simulink model "LUGOT"  (R2021a)
settings: Solver=FixedStepDiscrete  StartTime=0.0  StopTime=length(time_uwb)-1  FixedStep=Ts  MaxStep=Ts  RelTol=1e-3
values from neighbouring files (symbols this model uses):
  a = (vx .* ax + vy .* ay) ./ v    [relative_spd_vs_residual.m]    (also in smoothing_spline_fit.m)
  num_init_steps = uint8(3)    [main.m]
  outlier_threshold = standerd_deviation * 3.75 * 2 + 0.0    [main.m]
  Ts = 1.    (= 1)    [main.m]    (also in stateTransitionFcn_PF.m = 0.01)
undefined symbols (not defined in the file or in its folder): delta_h, Discrete, Time
libraries: sharedTrackingLibrary x9, simulink x6, dspstat3 x4, ctrlSharedLib x1
(part 1 of 2)
settings Model: Creator=bit202  LastModifiedBy=bit202
settings SolverCC: PositivePriorityOrder=on  AutoInsertRateTranBlk=on
settings DataIOCC: ReturnWorkspaceOutputs=off

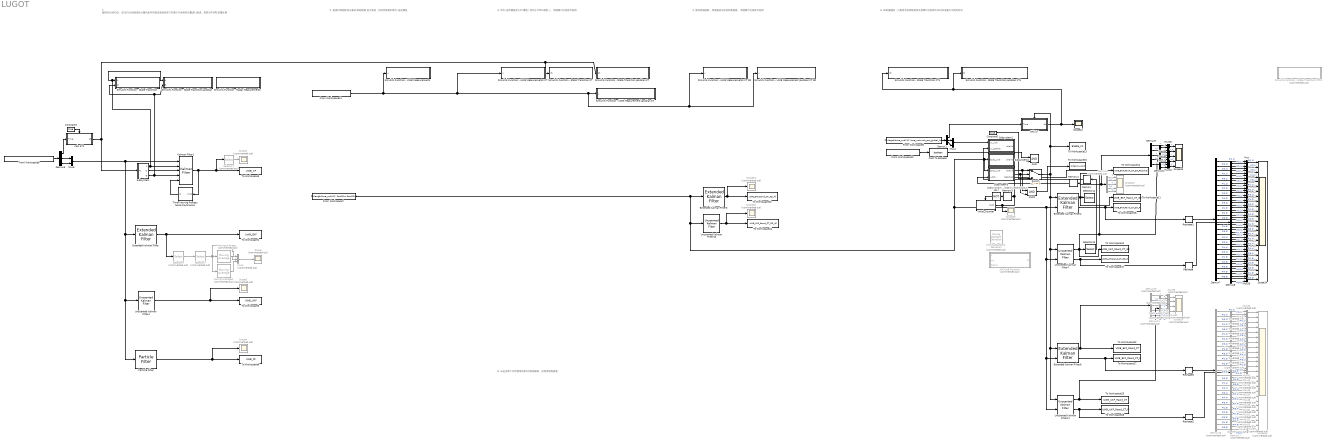
== system LUGOT ==
  note: 随着ΔT的变大，阈值可以考虑适当变大
  note: 1. 直接对分别对d1、d2进行分别滤波后计算的后车初始位姿坐标系下的笛卡尔坐标系位置进行滤波，把其当作GPS位置处理
  note: 2. 直接对观测标签与基站 原始距离 进行滤波，但仍然使用的是CV运动模型
  note: 3. 将CV运动模型改为CT模型（相当于CTRV模型）。
      | 观测雅可比矩阵不能用
  note: 4. 修改观测函数，考虑基站与标签的高度差。
      | 观测雅可比矩阵不能用
  note: 5. 异常值剔除，只是将状态转移矩阵及其雅可比矩阵的dt时间设置为不同的时间
  note: 6. 右边这两个仍然使用的是3的观测函数，没有考虑高度差
  AND : Logic  IconShape=distinctive  AllPortsSameDT=off  OutDataTypeStr=boolean
  AND1 : Logic  IconShape=distinctive  AllPortsSameDT=off  OutDataTypeStr=boolean
  Cast To Boolean : DataTypeConversion  OutDataTypeStr=boolean
  Constant1 : Constant  Value=true
  Constant3 : Constant  Value=true
  Demux1 : Demux  Outputs=3
  Demux10 : Demux  Outputs=5
  Demux11 : Demux  Commented=on  Outputs=5
  Demux16 : Demux  Commented=on  Outputs=25
  Demux17 : Demux  Commented=on  Outputs=25
  Demux18 : Demux  Commented=on  Outputs=5
  Demux3 : Demux  Outputs=3
  Demux4 : Demux  Commented=on  Outputs=5
  Demux7 : Demux  Outputs=25
  Demux8 : Demux  Outputs=25
  Demux9 : Demux  Outputs=5
  Extended Kalman Filter : sharedTrackingLibrary/Extended Kalman Filter  StateTransitionFcn=stateTransitionFcn  HasStateTransitionJacobianFcn=on  StateTransitionJacobianFcn=stateTransitionJacobianFcn  HasAdditiveProcessNoise=Nonadditive  ProcessNoise=[0.2 0; 0 0.2]  HasTimeVaryingProcessNoise=off  HasStateTransitionFcnExtraArgument=0  InitialState=[28; 0.001; 0.001; 0.001]  InitialStateCovariance=1  MeasurementFcn1=gpsMeasurementFcn  HasMeasurementJacobianFcn1=off  HasMeasurementEnablePort1=off  HasAdditiveMeasurementNoise1=Additive  MeasurementNoise1=[100 0; 0 100]  HasTimeVaryingMeasurementNoise1=off  HasMeasurementFcnExtraArgument1=0  MeasurementFcn2=myMeasurementFcn  HasMeasurementJacobianFcn2=off  HasMeasurementEnablePort2=off  HasAdditiveMeasurementNoise2=Additive  MeasurementNoise2=[0.0025 0; 0 0.0025]  HasTimeVaryingMeasurementNoise2=off  HasMeasurementFcnExtraArgument2=0  MeasurementFcn3=myMeasurementFcn  HasMeasurementJacobianFcn3=off  HasMeasurementEnablePort3=off  HasAdditiveMeasurementNoise3=Additive  MeasurementNoise3=1  HasTimeVaryingMeasurementNoise3=off  HasMeasurementFcnExtraArgument3=0  MeasurementFcn4=myMeasurementFcn  HasMeasurementJacobianFcn4=off  HasMeasurementEnablePort4=off  HasAdditiveMeasurementNoise4=Additive  MeasurementNoise4=1  HasTimeVaryingMeasurementNoise4=off  HasMeasurementFcnExtraArgument4=0  MeasurementFcn5=myMeasurementFcn  HasMeasurementJacobianFcn5=off  HasMeasurementEnablePort5=off  HasAdditiveMeasurementNoise5=Additive  MeasurementNoise5=1  HasTimeVaryingMeasurementNoise5=off  HasMeasurementFcnExtraArgument5=0  EnableMultirate=on  StateTransitionFcnSampleTime=Ts  MeasurementFcn1SampleTime=Ts  MeasurementFcn2SampleTime=1  MeasurementFcn3SampleTime=1  MeasurementFcn4SampleTime=1  MeasurementFcn5SampleTime=1  UseCurrentEstimator=on  OutputStateCovariance=off  DataType=double  SampleTime=0.01  NumberOfMeasurements=1
      settings: SourceProductBaseCode=CT,DR,TF,ID,LP,NV,AR,RO,RR,UV,VE
  Extended Kalman Filter2 : sharedTrackingLibrary/Extended Kalman Filter  StateTransitionFcn=stateTransitionCTEliminateFcn  HasStateTransitionJacobianFcn=on  StateTransitionJacobianFcn=stateTransitionJacobianCTFcn  HasAdditiveProcessNoise=Nonadditive  ProcessNoise=cov_process_noise  HasTimeVaryingProcessNoise=off  HasStateTransitionFcnExtraArgument=0  InitialState=init_state  InitialStateCovariance=0.5  MeasurementFcn1=uwbMeasurementCT3DFcn  HasMeasurementJacobianFcn1=off  MeasurementJacobianFcn1=uwbMeasurementJacobianCT3DFcn  HasMeasurementEnablePort1=on  HasAdditiveMeasurementNoise1=Additive  MeasurementNoise1=cov_measurement_noise  HasTimeVaryingMeasurementNoise1=off  HasMeasurementFcnExtraArgument1=0  MeasurementFcn2=myMeasurementFcn  HasMeasurementJacobianFcn2=off  HasMeasurementEnablePort2=off  HasAdditiveMeasurementNoise2=Additive  MeasurementNoise2=[0.0025 0; 0 0.0025]  HasTimeVaryingMeasurementNoise2=off  HasMeasurementFcnExtraArgument2=0  MeasurementFcn3=myMeasurementFcn  HasMeasurementJacobianFcn3=off  HasMeasurementEnablePort3=off  HasAdditiveMeasurementNoise3=Additive  MeasurementNoise3=1  HasTimeVaryingMeasurementNoise3=off  HasMeasurementFcnExtraArgument3=0  MeasurementFcn4=myMeasurementFcn  HasMeasurementJacobianFcn4=off  HasMeasurementEnablePort4=off  HasAdditiveMeasurementNoise4=Additive  MeasurementNoise4=1  HasTimeVaryingMeasurementNoise4=off  HasMeasurementFcnExtraArgument4=0  MeasurementFcn5=myMeasurementFcn  HasMeasurementJacobianFcn5=off  HasMeasurementEnablePort5=off  HasAdditiveMeasurementNoise5=Additive  MeasurementNoise5=1  HasTimeVaryingMeasurementNoise5=off  HasMeasurementFcnExtraArgument5=0  EnableMultirate=off  StateTransitionFcnSampleTime=0.01  MeasurementFcn1SampleTime=0.01  MeasurementFcn2SampleTime=1  MeasurementFcn3SampleTime=1  MeasurementFcn4SampleTime=1  MeasurementFcn5SampleTime=1  UseCurrentEstimator=on  OutputStateCovariance=on  DataType=double  SampleTime=Ts  NumberOfMeasurements=1
      settings: SourceProductBaseCode=CT,DR,TF,ID,LP,NV,AR,RO,RR,UV,VE
  Extended Kalman Filter5 : sharedTrackingLibrary/Extended Kalman Filter  StateTransitionFcn=stateTransitionCTFcn  HasStateTransitionJacobianFcn=on  StateTransitionJacobianFcn=stateTransitionJacobianCTFcn  HasAdditiveProcessNoise=Nonadditive  ProcessNoise=diag([0.2 0.2 0.2])  HasTimeVaryingProcessNoise=off  HasStateTransitionFcnExtraArgument=0  InitialState=init_state  InitialStateCovariance=0.5  MeasurementFcn1=uwbMeasurementCT3DFcn  HasMeasurementJacobianFcn1=off  MeasurementJacobianFcn1=uwbMeasurementJacobianCT3DFcn  HasMeasurementEnablePort1=off  HasAdditiveMeasurementNoise1=Additive  MeasurementNoise1=diag([1e-4 1e-4])  HasTimeVaryingMeasurementNoise1=off  HasMeasurementFcnExtraArgument1=0  MeasurementFcn2=myMeasurementFcn  HasMeasurementJacobianFcn2=off  HasMeasurementEnablePort2=off  HasAdditiveMeasurementNoise2=Additive  MeasurementNoise2=[0.0025 0; 0 0.0025]  HasTimeVaryingMeasurementNoise2=off  HasMeasurementFcnExtraArgument2=0  MeasurementFcn3=myMeasurementFcn  HasMeasurementJacobianFcn3=off  HasMeasurementEnablePort3=off  HasAdditiveMeasurementNoise3=Additive  MeasurementNoise3=1  HasTimeVaryingMeasurementNoise3=off  HasMeasurementFcnExtraArgument3=0  MeasurementFcn4=myMeasurementFcn  HasMeasurementJacobianFcn4=off  HasMeasurementEnablePort4=off  HasAdditiveMeasurementNoise4=Additive  MeasurementNoise4=1  HasTimeVaryingMeasurementNoise4=off  HasMeasurementFcnExtraArgument4=0  MeasurementFcn5=myMeasurementFcn  HasMeasurementJacobianFcn5=off  HasMeasurementEnablePort5=off  HasAdditiveMeasurementNoise5=Additive  MeasurementNoise5=1  HasTimeVaryingMeasurementNoise5=off  HasMeasurementFcnExtraArgument5=0  EnableMultirate=off  StateTransitionFcnSampleTime=0.01  MeasurementFcn1SampleTime=0.01  MeasurementFcn2SampleTime=1  MeasurementFcn3SampleTime=1  MeasurementFcn4SampleTime=1  MeasurementFcn5SampleTime=1  UseCurrentEstimator=on  OutputStateCovariance=off  DataType=double  SampleTime=Ts  NumberOfMeasurements=1
      settings: SourceProductBaseCode=CT,DR,TF,ID,LP,NV,AR,RO,RR,UV,VE
  Extended Kalman Filter6 : sharedTrackingLibrary/Extended Kalman Filter  StateTransitionFcn=stateTransitionCTEliminateFcn  HasStateTransitionJacobianFcn=on  StateTransitionJacobianFcn=stateTransitionJacobianCTFcn  HasAdditiveProcessNoise=Nonadditive  ProcessNoise=cov_process_noise  HasTimeVaryingProcessNoise=off  HasStateTransitionFcnExtraArgument=0  InitialState=init_state  InitialStateCovariance=0.5  MeasurementFcn1=uwbMeasurementCTFcn  HasMeasurementJacobianFcn1=off  MeasurementJacobianFcn1=uwbMeasurementJacobianCT3DFcn  HasMeasurementEnablePort1=on  HasAdditiveMeasurementNoise1=Additive  MeasurementNoise1=cov_measurement_noise  HasTimeVaryingMeasurementNoise1=off  HasMeasurementFcnExtraArgument1=0  MeasurementFcn2=myMeasurementFcn  HasMeasurementJacobianFcn2=off  HasMeasurementEnablePort2=off  HasAdditiveMeasurementNoise2=Additive  MeasurementNoise2=[0.0025 0; 0 0.0025]  HasTimeVaryingMeasurementNoise2=off  HasMeasurementFcnExtraArgument2=0  MeasurementFcn3=myMeasurementFcn  HasMeasurementJacobianFcn3=off  HasMeasurementEnablePort3=off  HasAdditiveMeasurementNoise3=Additive  MeasurementNoise3=1  HasTimeVaryingMeasurementNoise3=off  HasMeasurementFcnExtraArgument3=0  MeasurementFcn4=myMeasurementFcn  HasMeasurementJacobianFcn4=off  HasMeasurementEnablePort4=off  HasAdditiveMeasurementNoise4=Additive  MeasurementNoise4=1  HasTimeVaryingMeasurementNoise4=off  HasMeasurementFcnExtraArgument4=0  MeasurementFcn5=myMeasurementFcn  HasMeasurementJacobianFcn5=off  HasMeasurementEnablePort5=off  HasAdditiveMeasurementNoise5=Additive  MeasurementNoise5=1  HasTimeVaryingMeasurementNoise5=off  HasMeasurementFcnExtraArgument5=0  EnableMultirate=off  StateTransitionFcnSampleTime=0.01  MeasurementFcn1SampleTime=0.01  MeasurementFcn2SampleTime=1  MeasurementFcn3SampleTime=1  MeasurementFcn4SampleTime=1  MeasurementFcn5SampleTime=1  UseCurrentEstimator=on  OutputStateCovariance=on  DataType=double  SampleTime=Ts  NumberOfMeasurements=1
      settings: SourceProductBaseCode=CT,DR,TF,ID,LP,NV,AR,RO,RR,UV,VE
  From Workspace10 : FromWorkspace  VariableName=[[0:length(time_uwb)-1].',valid_raw]  SampleTime=-1  Interpolate=off  OutputAfterFinalValue=Setting to zero
  From Workspace11 : FromWorkspace  VariableName=[[0:length(time_uwb)-1].',lidar_pos,theta]  SampleTime=-1  Interpolate=off  OutputAfterFinalValue=Setting to zero
  From Workspace7 : FromWorkspace  VariableName=[[0:length(time_uwb)-1].',RawD1m,RawD2m]  SampleTime=-1  Interpolate=off  OutputAfterFinalValue=Setting to zero
  From Workspace8 : FromWorkspace  VariableName=[[0:length(time_uwb)-1].',time_uwb,uwb_raw_global_lidar]  SampleTime=-1  Interpolate=off  OutputAfterFinalValue=Setting to zero
  From Workspace9 : FromWorkspace  VariableName=[[0:length(time_uwb)-1].',time_uwb,uwb_global_lidar]  SampleTime=-1
  Kalman Filter1 : ctrlSharedLib/Kalman Filter  TimeDomain=Discrete-Time  UseCurrentEstimator=on  ModelSource=Input port  ModelSourceVariable=ss(0.95,1,1,0,1)  A=[1 0 Ts 0; 0 1 0 Ts; 0 0 1 0; 0 0 0 1]  B=1  C=[1 0 0 0; 0 1 0 0]  D=0  NumberOfStates=4  NumberOfInputs=2  NumberOfOutputs=2  InitialEstimateSource=Dialog  X0=[28; 0.001; 0.001; 0.001]  P0=diag([10 10 10 10])  UseK=off  UseGH=on  NumberOfProcessNoiseInputs=1  G=[Ts/2 0; 0 Ts/2; 1 0; 0 1]  TimeInvariantG=off  H=diag([0 0])  TimeInvariantH=on  Q=[0.05 0; 0 0.05]  TimeInvariantQ=off  R=diag([50 50])  TimeInvariantR=on  N=0  TimeInvariantN=on  AddInputPort=off  AddEnablePort=off  OutputEstimatedY=off  OutputP=off  Ts=-1
  MATLAB Function : MATLAB Function  Commented=on  TreatAsAtomicUnit=on
  Memory : Memory  InitialCondition=[25, 0]  InheritSampleTime=on
  Memory1 : Memory  InitialCondition=[28; 0.2; 0.01; 0.2; 0.001]  InheritSampleTime=on
  Memory3 : Memory  InheritSampleTime=on
  Moving Average : dspstat3/Moving Average  Commented=on  Method=Sliding window  ForgettingFactorPort=off  SpecifyWindowLength=on  WindowLength=20  ForgettingFactor=0.9  SimulateUsing=Code generation
  Moving Average2 : dspstat3/Moving Average  Commented=on  Method=Exponential weighting  ForgettingFactorPort=off  SpecifyWindowLength=on  WindowLength=20  ForgettingFactor=0.95  SimulateUsing=Code generation
  Moving Standard Deviation : dspstat3/Moving Standard Deviation  Commented=on  Method=Sliding window  ForgettingFactorPort=off  SpecifyWindowLength=on  WindowLength=20  ForgettingFactor=0.9  SimulateUsing=Code generation
      settings: SourceProductBaseCode=DS
  Mux{,4..34} (32 alike) : Mux  Inputs=2
  Mux2 : Mux  Commented=on  Inputs=3
  Mux{35..64} (30 alike) : Mux  Commented=on  Inputs=2
  NOT : Logic  Operator=NOT  IconShape=distinctive  AllPortsSameDT=off  OutDataTypeStr=boolean
  Particle Filter : sharedTrackingLibrary/Particle Filter  StateTransitionFcn=stateTransitionFcn_PF  HasStateTransitionFcnExtraArgument=0  NumberOfParticles=100  InitialDistribution=Gaussian  InitialMean=[28; 0.001; 0.001; 0.001]  InitialCovariance=diag([0.2 0.2 0.2 0.2])  InitialStateBounds=[-3 3; -3 3]  InitialParticles=[]  InitialWeights=[]  CircularVariables=0  StateOrientation=Column  MeasurementLikelihoodFcn1=gpsMeasurementLikelihoodFcn  HasMeasurementEnablePort1=off  HasMeasurementFcnExtraArgument1=0  HasMeasurementEnablePort2=off  HasMeasurementFcnExtraArgument2=0  HasMeasurementEnablePort3=off  HasMeasurementFcnExtraArgument3=0  HasMeasurementEnablePort4=off  HasMeasurementFcnExtraArgument4=0  HasMeasurementEnablePort5=off  HasMeasurementFcnExtraArgument5=0  ResamplingMethod=Multinomial  TriggerMethod=Ratio  MinEffectiveParticleRatio=0.5  SamplingInterval=1  Randomness=Repeatable  Seed=0  StateEstimationMethod=Mean  OutputParticles=off  OutputWeights=off  OutputStateCovariance=off  UseCurrentEstimator=on  EnableMultirate=off  StateTransitionFcnSampleTime=1  MeasurementLikelihoodFcn1SampleTime=1  MeasurementLikelihoodFcn2SampleTime=1  MeasurementLikelihoodFcn3SampleTime=1  MeasurementLikelihoodFcn4SampleTime=1  MeasurementLikelihoodFcn5SampleTime=1  DataType=double  SampleTime=Ts  NumberOfMeasurements=1
      settings: SourceProductBaseCode=CT,DR,TF,ID,LP,NV,AR,RO,RR,UV,VE
  Reshape{,1..3} (4 alike) : Reshape
  Scope{,1,3..4,18..19,28} (7 alike) : Scope  Commented=on
  Scope10 : Scope  Commented=on  NumInputPorts=5
  Scope12 : Scope
  Scope14 : Scope  NumInputPorts=25
  Scope15 : Scope  NumInputPorts=5
  Scope23 : Scope  Commented=on  NumInputPorts=25
  Scope24 : Scope  Commented=on  NumInputPorts=5
  Selector13 : Selector  InputPortWidth=5  IndexOptions=Index vector (dialog)  Indices=[1 3]  OutputSizes=1
  Selector14 : Selector  InputPortWidth=5  IndexOptions=Index vector (dialog)  Indices=[1 3]  OutputSizes=1
  Selector2 : Selector  Commented=on  InputPortWidth=2  IndexOptions=Index vector (dialog)  Indices=1  OutputSizes=1
  Selector7 : Selector  Commented=on  InputPortWidth=4  IndexOptions=Index vector (dialog)  Indices=[1 2]  OutputSizes=1
  Selector9 : Selector  Commented=on  InputPortWidth=4  IndexOptions=Index vector (dialog)  Indices=[1 2]  OutputSizes=1
  Simulink Function - Radar Measurements : Subsystem  TreatAsAtomicUnit=on
  Simulink Function - State Transition : Subsystem  TreatAsAtomicUnit=on
  Simulink Function - State Transition CT : Subsystem  TreatAsAtomicUnit=on
  Simulink Function - State Transition CT1 : Subsystem  TreatAsAtomicUnit=on
  Simulink Function - State Transition CTRV : Subsystem  Commented=on  TreatAsAtomicUnit=on
  Simulink Function - State Transition Jacobian : Subsystem  TreatAsAtomicUnit=on
  Simulink Function - State Transition Jacobian CT : Subsystem  TreatAsAtomicUnit=on
  Simulink Function - State Transition Jacobian CT1 : Subsystem  TreatAsAtomicUnit=on
  Simulink Function - UWB Measurement Jacobian CT : Subsystem  TreatAsAtomicUnit=on
  Simulink Function - UWB Measurement Jacobian CT 3D : Subsystem  TreatAsAtomicUnit=on
  Simulink Function - UWB Measurements : Subsystem  TreatAsAtomicUnit=on
  Simulink Function - UWB Measurements CT : Subsystem  TreatAsAtomicUnit=on
  Simulink Function - UWB Measurements CT 3D : Subsystem  TreatAsAtomicUnit=on
  Subsystem : Subsystem
  Subsystem1 : Subsystem
  Subsystem2 : Subsystem
  Subsystem3 : Subsystem
  Switch : Switch  Criteria=u2 ~= 0
  Time-Varying Process Noise Covariance : Subsystem
  To Workspace1 : ToWorkspace  VariableName=UWB_EKF  SaveFormat=Structure With Time  SampleTime=-1
  To Workspace11 : ToWorkspace  VariableName=UWB_EKF_Rawd_CT_3D  SaveFormat=Structure With Time  SampleTime=-1
  To Workspace12 : ToWorkspace  VariableName=UWB_UKF_Rawd_CT_3D  SaveFormat=Structure With Time  SampleTime=-1
  To Workspace13 : ToWorkspace  VariableName=Enable_KF  SaveFormat=Structure With Time  SampleTime=-1
  To Workspace14 : ToWorkspace  VariableName=UWB_EKF_Rawd_CT_3D_Residual  SaveFormat=Structure With Time  SampleTime=-1
  To Workspace15 : ToWorkspace  VariableName=criterion_valid  SaveFormat=Structure With Time  SampleTime=-1
  To Workspace16 : ToWorkspace  VariableName=UWB_EKF_Rawd_CT_3D_P  SaveFormat=Structure With Time  SampleTime=-1
  To Workspace17 : ToWorkspace  VariableName=UWB_UKF_Rawd_CT_3D_P  SaveFormat=Structure With Time  SampleTime=-1
  To Workspace20 : ToWorkspace  VariableName=UWB_EKF_Rawd_CT_3D_All  SaveFormat=Structure With Time  SampleTime=-1
  To Workspace21 : ToWorkspace  VariableName=UWB_UKF_Rawd_CT_3D_All  SaveFormat=Structure With Time  SampleTime=-1
  To Workspace22 : ToWorkspace  VariableName=UWB_EKF_Rawd_CT  SaveFormat=Structure With Time  SampleTime=-1
  To Workspace23 : ToWorkspace  VariableName=UWB_UKF_Rawd_CT  SaveFormat=Structure With Time  SampleTime=-1
  To Workspace27 : ToWorkspace  VariableName=UWB_EKF_Rawd_CT_P  SaveFormat=Structure With Time  SampleTime=-1
  To Workspace28 : ToWorkspace  VariableName=UWB_UKF_Rawd_CT_P  SaveFormat=Structure With Time  SampleTime=-1
  To Workspace3 : ToWorkspace  VariableName=UWB_KF  SaveFormat=Structure With Time  SampleTime=-1
  To Workspace5 : ToWorkspace  VariableName=UWB_UKF  SaveFormat=Structure With Time  SampleTime=-1
  To Workspace6 : ToWorkspace  VariableName=UWB_PF  SaveFormat=Structure With Time  SampleTime=-1
  Unscented Kalman Filter10 : sharedTrackingLibrary/Unscented Kalman Filter  StateTransitionFcn=stateTransitionCTFcn  HasAdditiveProcessNoise=Nonadditive  ProcessNoise=diag([0.2 0.2 0.2])  HasTimeVaryingProcessNoise=off  HasStateTransitionFcnExtraArgument=0  InitialState=init_state  InitialStateCovariance=0.5  Alpha=1e-3  Beta=2  Kappa=0  MeasurementFcn1=uwbMeasurementCT3DFcn  HasMeasurementEnablePort1=off  HasAdditiveMeasurementNoise1=Additive  MeasurementNoise1=diag([1e-4 1e-4])  HasTimeVaryingMeasurementNoise1=off  HasMeasurementFcnExtraArgument1=0  MeasurementFcn2=myMeasurementFcn  HasMeasurementEnablePort2=off  HasAdditiveMeasurementNoise2=Additive  MeasurementNoise2=1  HasTimeVaryingMeasurementNoise2=off  HasMeasurementFcnExtraArgument2=0  MeasurementFcn3=myMeasurementFcn  HasMeasurementEnablePort3=off  HasAdditiveMeasurementNoise3=Additive  MeasurementNoise3=1  HasTimeVaryingMeasurementNoise3=off  HasMeasurementFcnExtraArgument3=0  MeasurementFcn4=myMeasurementFcn  HasMeasurementEnablePort4=off  HasAdditiveMeasurementNoise4=Additive  MeasurementNoise4=1  HasTimeVaryingMeasurementNoise4=off  HasMeasurementFcnExtraArgument4=0  MeasurementFcn5=myMeasurementFcn  HasMeasurementEnablePort5=off  HasAdditiveMeasurementNoise5=Additive  MeasurementNoise5=1  HasTimeVaryingMeasurementNoise5=off  HasMeasurementFcnExtraArgument5=0  EnableMultirate=off  StateTransitionFcnSampleTime=1  MeasurementFcn1SampleTime=1  MeasurementFcn2SampleTime=1  MeasurementFcn3SampleTime=1  MeasurementFcn4SampleTime=1  MeasurementFcn5SampleTime=1  UseCurrentEstimator=on  OutputStateCovariance=off  DataType=double  SampleTime=Ts  NumberOfMeasurements=1
      settings: SourceProductBaseCode=CT,DR,TF,ID,LP,NV,AR,RO,RR,UV,VE
  Unscented Kalman Filter11 : sharedTrackingLibrary/Unscented Kalman Filter  StateTransitionFcn=stateTransitionCTEliminateFcn  HasAdditiveProcessNoise=Nonadditive  ProcessNoise=cov_process_noise  HasTimeVaryingProcessNoise=off  HasStateTransitionFcnExtraArgument=0  InitialState=init_state  InitialStateCovariance=0.5  Alpha=1e-1  Beta=2  Kappa=3  MeasurementFcn1=uwbMeasurementCTFcn  HasMeasurementEnablePort1=on  HasAdditiveMeasurementNoise1=Additive  MeasurementNoise1=cov_measurement_noise  HasTimeVaryingMeasurementNoise1=off  HasMeasurementFcnExtraArgument1=0  MeasurementFcn2=myMeasurementFcn  HasMeasurementEnablePort2=off  HasAdditiveMeasurementNoise2=Additive  MeasurementNoise2=1  HasTimeVaryingMeasurementNoise2=off  HasMeasurementFcnExtraArgument2=0  MeasurementFcn3=myMeasurementFcn  HasMeasurementEnablePort3=off  HasAdditiveMeasurementNoise3=Additive  MeasurementNoise3=1  HasTimeVaryingMeasurementNoise3=off  HasMeasurementFcnExtraArgument3=0  MeasurementFcn4=myMeasurementFcn  HasMeasurementEnablePort4=off  HasAdditiveMeasurementNoise4=Additive  MeasurementNoise4=1  HasTimeVaryingMeasurementNoise4=off  HasMeasurementFcnExtraArgument4=0  MeasurementFcn5=myMeasurementFcn  HasMeasurementEnablePort5=off  HasAdditiveMeasurementNoise5=Additive  MeasurementNoise5=1  HasTimeVaryingMeasurementNoise5=off  HasMeasurementFcnExtraArgument5=0  EnableMultirate=off  StateTransitionFcnSampleTime=1  MeasurementFcn1SampleTime=1  MeasurementFcn2SampleTime=1  MeasurementFcn3SampleTime=1  MeasurementFcn4SampleTime=1  MeasurementFcn5SampleTime=1  UseCurrentEstimator=on  OutputStateCovariance=on  DataType=double  SampleTime=Ts  NumberOfMeasurements=1
      settings: SourceProductBaseCode=CT,DR,TF,ID,LP,NV,AR,RO,RR,UV,VE
  Unscented Kalman Filter4 : sharedTrackingLibrary/Unscented Kalman Filter  StateTransitionFcn=stateTransitionFcn  HasAdditiveProcessNoise=Nonadditive  ProcessNoise=[0.2 0; 0 0.2]  HasTimeVaryingProcessNoise=off  HasStateTransitionFcnExtraArgument=0  InitialState=[28; 0.001; 0.001; 0.001]  InitialStateCovariance=0.5  Alpha=1e-3  Beta=2  Kappa=0  MeasurementFcn1=gpsMeasurementFcn  HasMeasurementEnablePort1=off  HasAdditiveMeasurementNoise1=Additive  MeasurementNoise1=[100 0; 0 100]  HasTimeVaryingMeasurementNoise1=off  HasMeasurementFcnExtraArgument1=0  MeasurementFcn2=myMeasurementFcn  HasMeasurementEnablePort2=off  HasAdditiveMeasurementNoise2=Additive  MeasurementNoise2=1  HasTimeVaryingMeasurementNoise2=off  HasMeasurementFcnExtraArgument2=0  MeasurementFcn3=myMeasurementFcn  HasMeasurementEnablePort3=off  HasAdditiveMeasurementNoise3=Additive  MeasurementNoise3=1  HasTimeVaryingMeasurementNoise3=off  HasMeasurementFcnExtraArgument3=0  MeasurementFcn4=myMeasurementFcn  HasMeasurementEnablePort4=off  HasAdditiveMeasurementNoise4=Additive  MeasurementNoise4=1  HasTimeVaryingMeasurementNoise4=off  HasMeasurementFcnExtraArgument4=0  MeasurementFcn5=myMeasurementFcn  HasMeasurementEnablePort5=off  HasAdditiveMeasurementNoise5=Additive  MeasurementNoise5=1  HasTimeVaryingMeasurementNoise5=off  HasMeasurementFcnExtraArgument5=0  EnableMultirate=off  StateTransitionFcnSampleTime=1  MeasurementFcn1SampleTime=1  MeasurementFcn2SampleTime=1  MeasurementFcn3SampleTime=1  MeasurementFcn4SampleTime=1  MeasurementFcn5SampleTime=1  UseCurrentEstimator=on  OutputStateCovariance=off  DataType=double  SampleTime=Ts  NumberOfMeasurements=1
      settings: SourceProductBaseCode=CT,DR,TF,ID,LP,NV,AR,RO,RR,UV,VE
  Unscented Kalman Filter7 : sharedTrackingLibrary/Unscented Kalman Filter  StateTransitionFcn=stateTransitionCTEliminateFcn  HasAdditiveProcessNoise=Nonadditive  ProcessNoise=cov_process_noise  HasTimeVaryingProcessNoise=off  HasStateTransitionFcnExtraArgument=0  InitialState=init_state  InitialStateCovariance=0.5  Alpha=1e-1  Beta=2  Kappa=3  MeasurementFcn1=uwbMeasurementCT3DFcn  HasMeasurementEnablePort1=on  HasAdditiveMeasurementNoise1=Additive  MeasurementNoise1=cov_measurement_noise  HasTimeVaryingMeasurementNoise1=off  HasMeasurementFcnExtraArgument1=0  MeasurementFcn2=myMeasurementFcn  HasMeasurementEnablePort2=off  HasAdditiveMeasurementNoise2=Additive  MeasurementNoise2=1  HasTimeVaryingMeasurementNoise2=off  HasMeasurementFcnExtraArgument2=0  MeasurementFcn3=myMeasurementFcn  HasMeasurementEnablePort3=off  HasAdditiveMeasurementNoise3=Additive  MeasurementNoise3=1  HasTimeVaryingMeasurementNoise3=off  HasMeasurementFcnExtraArgument3=0  MeasurementFcn4=myMeasurementFcn  HasMeasurementEnablePort4=off  HasAdditiveMeasurementNoise4=Additive  MeasurementNoise4=1  HasTimeVaryingMeasurementNoise4=off  HasMeasurementFcnExtraArgument4=0  MeasurementFcn5=myMeasurementFcn  HasMeasurementEnablePort5=off  HasAdditiveMeasurementNoise5=Additive  MeasurementNoise5=1  HasTimeVaryingMeasurementNoise5=off  HasMeasurementFcnExtraArgument5=0  EnableMultirate=off  StateTransitionFcnSampleTime=1  MeasurementFcn1SampleTime=1  MeasurementFcn2SampleTime=1  MeasurementFcn3SampleTime=1  MeasurementFcn4SampleTime=1  MeasurementFcn5SampleTime=1  UseCurrentEstimator=on  OutputStateCovariance=on  DataType=double  SampleTime=Ts  NumberOfMeasurements=1
      settings: SourceProductBaseCode=CT,DR,TF,ID,LP,NV,AR,RO,RR,UV,VE
  calc ΔT : Subsystem  TreatAsAtomicUnit=on
  calc ΔT1 : Subsystem  TreatAsAtomicUnit=on
  initial_counter : Subsystem
  wires:
  Mux6/1 -> Particle Filter/1, Unscented Kalman Filter4/1, Extended Kalman Filter/1, Kalman Filter1/1
  Selector2/1 -> Moving Average2/1, Mux2/1, Moving Average/1
  Extended Kalman Filter/1 -> Selector9/1, To Workspace1/1
  Moving Average/1 -> Mux2/2
  Mux2/1 -> Scope/1
  Moving Average2/1 -> Mux2/3
  Kalman Filter1/1 -> To Workspace3/1, Selector7/1, Time-Varying Process Noise Covariance/1(xhat)
  Selector7/1 -> Scope1/1
  Time-Varying Process Noise Covariance/1(Q) -> Kalman Filter1/5
  Unscented Kalman Filter4/1 -> To Workspace5/1, Scope3/1
  Selector9/1 -> Selector2/1
  Particle Filter/1 -> Scope4/1, To Workspace6/1
  From Workspace11/1 -> Simulink Function - UWB Measurements/1(u), Simulink Function - UWB Measurements CT/1(u), Simulink Function - UWB Measurement Jacobian CT 3D/1(u), Simulink Function - UWB Measurements CT 3D/1(u), Simulink Function - UWB Measurement Jacobian CT/1(u)
  Selector13/1 -> Memory/1
  Demux1/2 -> Mux4/1
  Demux1/3 -> Mux4/2
  Demux1/1 -> calc ΔT/1(Time)
  Demux3/2 -> Mux6/1
  Demux3/3 -> Mux6/2
  Demux3/1 -> calc ΔT1/1(Time)
  Constant3/1 -> calc ΔT1/Enable
  From Workspace8/1 -> Demux1/1
  Subsystem/3(G) -> Kalman Filter1/4, Simulink Function - State Transition Jacobian/2(G), Simulink Function - State Transition/2(G)
  Subsystem/1(A) -> Kalman Filter1/2, Simulink Function - State Transition Jacobian/1(A), Simulink Function - State Transition/1(A)
  Subsystem/2(C) -> Kalman Filter1/3
  Demux4/1 -> Scope10/1  "x"
  Demux4/2 -> Scope10/2  "v_x"
  Demux4/3 -> Scope10/3  "y"
  Demux4/4 -> Scope10/4  "v_y"
  Demux4/5 -> Scope10/5  "ω"
  calc ΔT/1(dt) -> Scope12/1, Simulink Function - State Transition Jacobian CT1/1(dt), Simulink Function - State Transition CT1/1(dt)
  calc ΔT1/1(dt) -> Subsystem/1(Ts), Simulink Function - State Transition CT/1(dt), Simulink Function - State Transition Jacobian CT/1(dt)
  From Workspace10/1 -> Cast To Boolean/1
  Mux4/1 -> Subsystem1/1(xy_uwb)
  Memory/1 -> Subsystem1/2(xy_predict)
  Subsystem2/1(isValid) -> AND/2
  Cast To Boolean/1 -> AND/1
  Memory1/1 -> Subsystem3/2(x_hat)
  Subsystem3/2(Residual) -> To Workspace14/1
  Extended Kalman Filter2/2 -> Reshape1/1, To Workspace16/1
  Unscented Kalman Filter7/2 -> To Workspace17/1, Reshape/1
  Mux/1 -> Scope14/1  "P(1,1)"
  Mux5/1 -> Scope14/2  "P(2,1)"
  Mux7/1 -> Scope14/3  "P(3,1)"
  Mux8/1 -> Scope14/4  "P(4,1)"
  Mux9/1 -> Scope14/5  "P(5,1)"
  Mux10/1 -> Scope14/6  "P(1,2)"
  Mux11/1 -> Scope14/7  "P(2,2)"
  Mux12/1 -> Scope14/8  "P(3,2)"
  Mux13/1 -> Scope14/9  "P(4,2)"
  Mux14/1 -> Scope14/10  "P(5,2)"
  Mux15/1 -> Scope14/11  "P(1,3)"
  Mux16/1 -> Scope14/12  "P(2,3)"
  Mux17/1 -> Scope14/13  "P(3,3)"
  Mux18/1 -> Scope14/14  "P(4,3)"
  Mux19/1 -> Scope14/15  "P(5,3)"
  Mux20/1 -> Scope14/16  "P(1,4)"
  Mux21/1 -> Scope14/17  "P(2,4)"
  Mux22/1 -> Scope14/18  "P(3,4)"
  Mux23/1 -> Scope14/19  "P(4,4)"
  Mux24/1 -> Scope14/20  "P(5,4)"
  Mux25/1 -> Scope14/21  "P(1,5)"
  Mux26/1 -> Scope14/22  "P(2,5)"
  Mux27/1 -> Scope14/23  "P(3,5)"
  Mux28/1 -> Scope14/24  "P(4,5)"
  Mux29/1 -> Scope14/25  "P(5,5)"
  Reshape1/1 -> Demux7/1
  Demux7/19 -> Mux23/1  "P(4,4)"
  Demux7/12 -> Mux16/1  "P(2,3)"
  Demux7/20 -> Mux24/1  "P(5,4)"
  Demux7/2 -> Mux5/1  "P(2,1)"
  Demux7/1 -> Mux/1  "P(1,1)"
  Demux7/25 -> Mux29/1  "P(5,5)"
  Demux7/21 -> Mux25/1  "P(1,5)"
  Demux7/22 -> Mux26/1  "P(2,5)"
  Demux7/23 -> Mux27/1  "P(3,5)"
  Demux7/24 -> Mux28/1  "P(4,5)"
  Demux7/9 -> Mux13/1  "P(4,2)"
  Demux7/3 -> Mux7/1  "P(3,1)"
  Demux7/6 -> Mux10/1  "P(1,2)"
  Demux7/17 -> Mux21/1  "P(2,4)"
  Demux7/11 -> Mux15/1  "P(1,3)"
  Demux7/8 -> Mux12/1  "P(3,2)"
  Demux7/5 -> Mux9/1  "P(5,1)"
  Demux7/4 -> Mux8/1  "P(4,1)"
  Demux7/10 -> Mux14/1  "P(5,2)"
  Demux7/18 -> Mux22/1  "P(3,4)"
  Demux7/14 -> Mux18/1  "P(4,3)"
  Demux7/7 -> Mux11/1  "P(2,2)"
  Demux7/15 -> Mux19/1  "P(5,3)"
  Demux7/13 -> Mux17/1  "P(3,3)"
  Demux7/16 -> Mux20/1  "P(1,4)"
  Demux8/6 -> Mux10/2  "P(1,2)"
  Demux8/7 -> Mux11/2  "P(2,2)"
  Demux8/1 -> Mux/2  "P(1,1)"
  Reshape/1 -> Demux8/1
  Demux8/22 -> Mux26/2  "P(2,5)"
  Demux8/2 -> Mux5/2  "P(2,1)"
  Demux8/8 -> Mux12/2  "P(3,2)"
  Demux8/14 -> Mux18/2  "P(4,3)"
  Demux8/13 -> Mux17/2  "P(3,3)"
  Demux8/5 -> Mux9/2  "P(5,1)"
  Demux8/23 -> Mux27/2  "P(3,5)"
  Demux8/4 -> Mux8/2  "P(4,1)"
  Demux8/11 -> Mux15/2  "P(1,3)"
  Demux8/25 -> Mux29/2  "P(5,5)"
  Demux8/9 -> Mux13/2  "P(4,2)"
  Demux8/20 -> Mux24/2  "P(5,4)"
  Demux8/10 -> Mux14/2  "P(5,2)"
  Demux8/24 -> Mux28/2  "P(4,5)"
  Demux8/15 -> Mux19/2  "P(5,3)"
  Demux8/3 -> Mux7/2  "P(3,1)"
  Demux8/16 -> Mux20/2  "P(1,4)"
  Demux8/12 -> Mux16/2  "P(2,3)"
  Demux8/21 -> Mux25/2  "P(1,5)"
  Demux8/18 -> Mux22/2  "P(3,4)"
  Demux8/17 -> Mux21/2  "P(2,4)"
  Demux8/19 -> Mux23/2  "P(4,4)"
  Mux30/1 -> Scope15/1  "x"
  Mux31/1 -> Scope15/2  "v_x"
  Mux32/1 -> Scope15/3  "y"
  Mux33/1 -> Scope15/4  "v_y"
  Mux34/1 -> Scope15/5  "ω"
  Demux9/5 -> Mux34/1  "ω"
  Demux9/4 -> Mux33/1  "v_y"
  Demux9/2 -> Mux31/1  "v_x"
  Demux9/3 -> Mux32/1  "y"
  Demux9/1 -> Mux30/1  "x"
  Extended Kalman Filter2/1 -> To Workspace11/1, Demux9/1, Demux4/1, Selector14/1
  Demux10/5 -> Mux34/2  "ω"
  Demux10/1 -> Mux30/2  "x"
  Demux10/3 -> Mux32/2  "y"
  Demux10/4 -> Mux33/2  "v_y"
  Demux10/2 -> Mux31/2  "v_x"
  Unscented Kalman Filter10/1 -> Scope18/1, To Workspace21/1
  Extended Kalman Filter5/1 -> To Workspace20/1, Scope19/1
  From Workspace7/1 -> Subsystem3/1(d1d2_uwb), Subsystem2/1(d1d2_uwb), Extended Kalman Filter6/2, Unscented Kalman Filter11/2, Unscented Kalman Filter7/2, Extended Kalman Filter2/2, Unscented Kalman Filter10/1, Extended Kalman Filter5/1
  Demux11/2 -> Mux57/2  "v_x"
  Demux11/4 -> Mux59/2  "v_y"
  Demux11/3 -> Mux58/2  "y"
  Demux11/1 -> Mux56/2  "x"
  Demux11/5 -> Mux60/2  "ω"
  Extended Kalman Filter6/1 -> Demux18/1, To Workspace22/1
  Demux18/1 -> Mux56/1  "x"
  Demux18/3 -> Mux58/1  "y"
  Demux18/2 -> Mux57/1  "v_x"
  Demux18/4 -> Mux59/1  "v_y"
  Demux18/5 -> Mux60/1  "ω"
  Mux60/1 -> Scope24/5
  Mux59/1 -> Scope24/4
  Mux58/1 -> Scope24/3
  Mux57/1 -> Scope24/2
  Mux56/1 -> Scope24/1
  Demux17/19 -> Mux49/2  "P(4,4)"
  Demux17/17 -> Mux47/2  "P(2,4)"
  Demux17/18 -> Mux48/2  "P(3,4)"
  Demux17/21 -> Mux51/2  "P(1,5)"
  Demux17/12 -> Mux42/2  "P(2,3)"
  Demux17/16 -> Mux46/2  "P(1,4)"
  Demux17/3 -> Mux62/2  "P(3,1)"
  Demux17/15 -> Mux45/2  "P(5,3)"
  Demux17/24 -> Mux54/2  "P(4,5)"
  Demux17/10 -> Mux40/2  "P(5,2)"
  Demux17/20 -> Mux50/2  "P(5,4)"
  Demux17/9 -> Mux39/2  "P(4,2)"
  Demux17/25 -> Mux55/2  "P(5,5)"
  Demux17/11 -> Mux41/2  "P(1,3)"
  Demux17/4 -> Mux63/2  "P(4,1)"
  Demux17/23 -> Mux53/2  "P(3,5)"
  Demux17/5 -> Mux64/2  "P(5,1)"
  Demux17/13 -> Mux43/2  "P(3,3)"
  Demux17/14 -> Mux44/2  "P(4,3)"
  Demux17/8 -> Mux38/2  "P(3,2)"
  Demux17/2 -> Mux61/2  "P(2,1)"
  Demux17/22 -> Mux52/2  "P(2,5)"
  Reshape2/1 -> Demux17/1
  Demux17/1 -> Mux35/2  "P(1,1)"
  Demux17/7 -> Mux37/2  "P(2,2)"
  Demux17/6 -> Mux36/2  "P(1,2)"
  Demux16/16 -> Mux46/1  "P(1,4)"
  Demux16/13 -> Mux43/1  "P(3,3)"
  Demux16/15 -> Mux45/1  "P(5,3)"
  Demux16/7 -> Mux37/1  "P(2,2)"
  Demux16/14 -> Mux44/1  "P(4,3)"
  Demux16/18 -> Mux48/1  "P(3,4)"
  Demux16/10 -> Mux40/1  "P(5,2)"
  Demux16/4 -> Mux63/1  "P(4,1)"
  Demux16/5 -> Mux64/1  "P(5,1)"
  Demux16/8 -> Mux38/1  "P(3,2)"
  Demux16/11 -> Mux41/1  "P(1,3)"
  Demux16/17 -> Mux47/1  "P(2,4)"
  Demux16/6 -> Mux36/1  "P(1,2)"
  Demux16/3 -> Mux62/1  "P(3,1)"
  Demux16/9 -> Mux39/1  "P(4,2)"
  Demux16/24 -> Mux54/1  "P(4,5)"
  Demux16/23 -> Mux53/1  "P(3,5)"
  Demux16/22 -> Mux52/1  "P(2,5)"
  Demux16/21 -> Mux51/1  "P(1,5)"
  Demux16/25 -> Mux55/1  "P(5,5)"
  Demux16/1 -> Mux35/1  "P(1,1)"
  Demux16/2 -> Mux61/1  "P(2,1)"
  Demux16/20 -> Mux50/1  "P(5,4)"
  Demux16/12 -> Mux42/1  "P(2,3)"
  Demux16/19 -> Mux49/1  "P(4,4)"
  Reshape3/1 -> Demux16/1
  Mux55/1 -> Scope23/25
  Mux54/1 -> Scope23/24
  Mux53/1 -> Scope23/23
  Mux52/1 -> Scope23/22
  Mux51/1 -> Scope23/21
  Mux50/1 -> Scope23/20
  Mux49/1 -> Scope23/19
  Mux48/1 -> Scope23/18
  Mux47/1 -> Scope23/17
  Mux46/1 -> Scope23/16
  Mux45/1 -> Scope23/15
  Mux44/1 -> Scope23/14
  Mux43/1 -> Scope23/13
  Mux42/1 -> Scope23/12
  Mux41/1 -> Scope23/11
  Mux40/1 -> Scope23/10
  Mux39/1 -> Scope23/9
  Mux38/1 -> Scope23/8
  Mux37/1 -> Scope23/7
  Mux36/1 -> Scope23/6
  Mux64/1 -> Scope23/5
  Mux63/1 -> Scope23/4
  Mux62/1 -> Scope23/3
  Mux61/1 -> Scope23/2
  Mux35/1 -> Scope23/1
  Unscented Kalman Filter11/2 -> Reshape2/1, To Workspace28/1
  Extended Kalman Filter6/2 -> To Workspace27/1, Reshape3/1
  Switch/1 -> calc ΔT/Enable, To Workspace13/1, Extended Kalman Filter6/1, Unscented Kalman Filter11/1, Unscented Kalman Filter7/1, Extended Kalman Filter2/1
  Unscented Kalman Filter11/1 -> Demux11/1, To Workspace23/1
  Unscented Kalman Filter7/1 -> To Workspace12/1, Selector13/1, Memory1/1, Demux10/1
  NOT/1 -> initial_counter/Enable
  initial_counter/1(Out1) -> AND1/2, Switch/2, Memory3/1, Scope28/1
  Memory3/1 -> NOT/1
  Constant1/1 -> Switch/3
  Subsystem3/1(isValid) -> AND1/1, Switch/1
  AND1/1 -> To Workspace15/1
  From Workspace9/1 -> Demux3/1

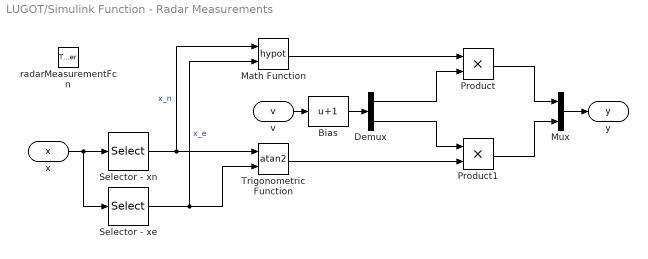
== system LUGOT/Simulink Function - Radar Measurements ==
  radarMeasurementFcn : TriggerPort  TriggerType=function-call  IsSimulinkFunction=on  FunctionName=radarMeasurementFcn  VariantControl=Variant
  Bias : Bias  Bias=1
  Demux : Demux  Outputs=2
  Math Function : Math  Operator=hypot  SignedPower=on  SaturateOnIntegerOverflow=on
  Mux : Mux  Inputs=2
  Product : Product
  Product1 : Product
  Selector - xe : Selector  InputPortWidth=4  IndexOptions=Index vector (dialog)  Indices=1  OutputSizes=1
  Selector - xn : Selector  InputPortWidth=4  IndexOptions=Index vector (dialog)  Indices=2  OutputSizes=1
  Trigonometric Function : Trigonometry  Operator=atan2
  x : ArgIn  DisableCoverage=on  PortDimensions=4  ArgumentName=x
  v : ArgIn  DisableCoverage=on  Port=2  PortDimensions=2  ArgumentName=v
  y : ArgOut  DisableCoverage=on  PortDimensions=2  ArgumentName=y
  wires:
  Mux/1 -> y/1
  x/1 -> Selector - xe/1, Selector - xn/1
  Selector - xn/1 -> Math Function/1, Trigonometric Function/1  "x_n"
  Selector - xe/1 -> Math Function/2, Trigonometric Function/2  "x_e"
  Trigonometric Function/1 -> Product1/2
  v/1 -> Bias/1
  Math Function/1 -> Product/1
  Product/1 -> Mux/1
  Product1/1 -> Mux/2
  Bias/1 -> Demux/1
  Demux/1 -> Product/2
  Demux/2 -> Product1/1

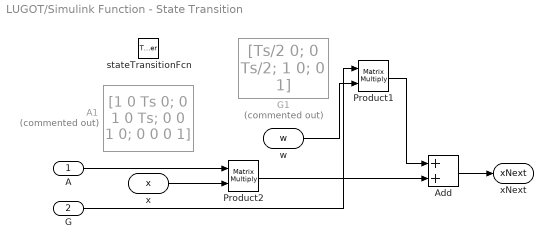
== system LUGOT/Simulink Function - State Transition ==
  A : Inport
  G : Inport  Port=2
  stateTransitionFcn : TriggerPort  TriggerType=function-call  IsSimulinkFunction=on  FunctionName=stateTransitionFcn  VariantControl=Variant
  A1 : Constant  Commented=on  Value=[1 0 Ts 0; 0 1 0 Ts; 0 0 1 0; 0 0 0 1]
  Add : Sum
  G1 : Constant  Commented=on  Value=[Ts/2 0; 0 Ts/2; 1 0; 0 1]
  Product1 : Product  Multiplication=Matrix(*)
  Product2 : Product  Multiplication=Matrix(*)
  x : ArgIn  DisableCoverage=on  PortDimensions=4  ArgumentName=x
  w : ArgIn  Port=2  PortDimensions=2  ArgumentName=w
  xNext : ArgOut  DisableCoverage=on  PortDimensions=4  ArgumentName=xNext
  wires:
  x/1 -> Product2/2
  A/1 -> Product2/1
  Product2/1 -> Add/2
  G/1 -> Product1/1
  w/1 -> Product1/2
  Product1/1 -> Add/1
  Add/1 -> xNext/1

== system LUGOT/Simulink Function - State Transition CT ==
  dt : Inport
  stateTransitionCTFcn : TriggerPort  TriggerType=function-call  IsSimulinkFunction=on  FunctionName=stateTransitionCTFcn  VariantControl=Variant
  MATLAB Function : MATLAB Function  TreatAsAtomicUnit=on
  x : ArgIn  DisableCoverage=on  PortDimensions=5  ArgumentName=x
  w : ArgIn  Port=2  PortDimensions=3  ArgumentName=w
  xNext : ArgOut  DisableCoverage=on  PortDimensions=5  ArgumentName=xNext
  wires:
  w/1 -> MATLAB Function/2(w)
  x/1 -> MATLAB Function/1(x)
  MATLAB Function/1(y) -> xNext/1
  dt/1 -> MATLAB Function/3(dt)

== system LUGOT/Simulink Function - State Transition CT1 ==
  dt : Inport
  stateTransitionCTEliminateFcn : TriggerPort  TriggerType=function-call  IsSimulinkFunction=on  FunctionName=stateTransitionCTEliminateFcn  VariantControl=Variant
  MATLAB Function : MATLAB Function  TreatAsAtomicUnit=on
  x : ArgIn  DisableCoverage=on  PortDimensions=5  ArgumentName=x
  w : ArgIn  Port=2  PortDimensions=3  ArgumentName=w
  xNext : ArgOut  DisableCoverage=on  PortDimensions=5  ArgumentName=xNext
  wires:
  dt/1 -> MATLAB Function/3(dt)
  MATLAB Function/1(y) -> xNext/1
  x/1 -> MATLAB Function/1(x)
  w/1 -> MATLAB Function/2(w)

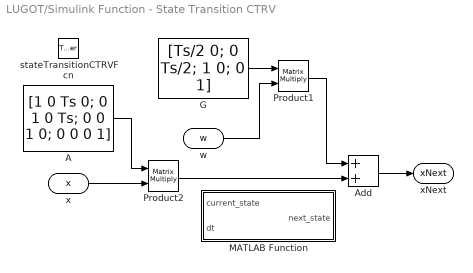
== system LUGOT/Simulink Function - State Transition CTRV ==
  stateTransitionCTRVFcn : TriggerPort  TriggerType=function-call  IsSimulinkFunction=on  FunctionName=stateTransitionCTRVFcn  VariantControl=Variant
  A : Constant  Value=[1 0 Ts 0; 0 1 0 Ts; 0 0 1 0; 0 0 0 1]
  Add : Sum
  G : Constant  Value=[Ts/2 0; 0 Ts/2; 1 0; 0 1]
  MATLAB Function : MATLAB Function  TreatAsAtomicUnit=on
  Product1 : Product  Multiplication=Matrix(*)
  Product2 : Product  Multiplication=Matrix(*)
  x : ArgIn  DisableCoverage=on  PortDimensions=4  ArgumentName=x
  w : ArgIn  Port=2  PortDimensions=2  ArgumentName=w
  xNext : ArgOut  DisableCoverage=on  PortDimensions=4  ArgumentName=xNext
  wires:
  x/1 -> Product2/2
  A/1 -> Product2/1
  Product2/1 -> Add/2
  G/1 -> Product1/1
  w/1 -> Product1/2
  Product1/1 -> Add/1
  Add/1 -> xNext/1

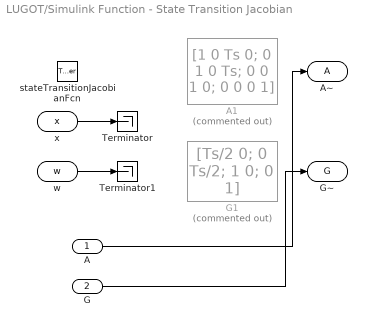
== system LUGOT/Simulink Function - State Transition Jacobian ==
  A : Inport
  G : Inport  Port=2
  stateTransitionJacobianFcn : TriggerPort  TriggerType=function-call  IsSimulinkFunction=on  FunctionName=stateTransitionJacobianFcn  VariantControl=Variant
  A1 : Constant  Commented=on  Value=[1 0 Ts 0; 0 1 0 Ts; 0 0 1 0; 0 0 0 1]
  G1 : Constant  Commented=on  Value=[Ts/2 0; 0 Ts/2; 1 0; 0 1]
  Terminator : Terminator
  Terminator1 : Terminator
  x : ArgIn  DisableCoverage=on  PortDimensions=4  ArgumentName=x
  w : ArgIn  Port=2  PortDimensions=2  ArgumentName=w
  A~ : ArgOut  DisableCoverage=on  PortDimensions=[4 4]  ArgumentName=A
  G~ : ArgOut  Port=2  PortDimensions=[4 2]  ArgumentName=G
  wires:
  G/1 -> G~/1
  x/1 -> Terminator/1
  w/1 -> Terminator1/1
  A/1 -> A~/1

== system LUGOT/Simulink Function - State Transition Jacobian CT ==
  dt : Inport
  stateTransitionJacobianCTFcn : TriggerPort  TriggerType=function-call  IsSimulinkFunction=on  FunctionName=stateTransitionJacobianCTFcn  VariantControl=Variant
  MATLAB Function : MATLAB Function  TreatAsAtomicUnit=on
  x : ArgIn  DisableCoverage=on  PortDimensions=5  ArgumentName=x
  w : ArgIn  Port=2  PortDimensions=3  ArgumentName=w
  A~ : ArgOut  DisableCoverage=on  PortDimensions=[5 5]  ArgumentName=A
  G~ : ArgOut  Port=2  PortDimensions=[5 3]  ArgumentName=G
  wires:
  MATLAB Function/1(A) -> A~/1
  w/1 -> MATLAB Function/2(w)
  x/1 -> MATLAB Function/1(x)
  MATLAB Function/2(G) -> G~/1
  dt/1 -> MATLAB Function/3(dt)

== system LUGOT/Simulink Function - State Transition Jacobian CT1 ==
  dt : Inport
  stateTransitionJacobianCTEliminateFcn : TriggerPort  TriggerType=function-call  IsSimulinkFunction=on  FunctionName=stateTransitionJacobianCTEliminateFcn  VariantControl=Variant
  MATLAB Function : MATLAB Function  TreatAsAtomicUnit=on
  x : ArgIn  DisableCoverage=on  PortDimensions=5  ArgumentName=x
  w : ArgIn  Port=2  PortDimensions=3  ArgumentName=w
  A : ArgOut  DisableCoverage=on  PortDimensions=[5 5]  ArgumentName=A
  G : ArgOut  Port=2  PortDimensions=[5 3]  ArgumentName=G
  wires:
  dt/1 -> MATLAB Function/3(dt)
  MATLAB Function/2(G) -> G/1
  x/1 -> MATLAB Function/1(x)
  w/1 -> MATLAB Function/2(w)
  MATLAB Function/1(A) -> A/1

== system LUGOT/Simulink Function - UWB Measurement Jacobian CT ==
  u : Inport
  uwbMeasurementJacobianCTFcn : TriggerPort  TriggerType=function-call  IsSimulinkFunction=on  FunctionName=uwbMeasurementJacobianCTFcn  VariantControl=Variant
  Constant : Constant  Value=a
  Demux : Demux  Outputs=3
  MATLAB Function : MATLAB Function  TreatAsAtomicUnit=on
  x : ArgIn  DisableCoverage=on  PortDimensions=5  ArgumentName=x
  C : ArgOut  DisableCoverage=on  PortDimensions=[2 5]  ArgumentName=C
  wires:
  x/1 -> MATLAB Function/1(X)
  MATLAB Function/1(H) -> C/1
  Constant/1 -> MATLAB Function/5(a)
  u/1 -> Demux/1
  Demux/1 -> MATLAB Function/2(x_ac)
  Demux/3 -> MATLAB Function/4(psi_ac)
  Demux/2 -> MATLAB Function/3(y_ac)

== system LUGOT/Simulink Function - UWB Measurement Jacobian CT 3D ==
  u : Inport
  uwbMeasurementJacobianCT3DFcn : TriggerPort  TriggerType=function-call  IsSimulinkFunction=on  FunctionName=uwbMeasurementJacobianCT3DFcn  VariantControl=Variant
  Constant : Constant  Value=a
  Constant1 : Constant  Value=delta_h
  Demux : Demux  Outputs=3
  MATLAB Function : MATLAB Function  TreatAsAtomicUnit=on
  x : ArgIn  DisableCoverage=on  PortDimensions=5  ArgumentName=x
  C : ArgOut  DisableCoverage=on  PortDimensions=[2 5]  ArgumentName=C
  wires:
  x/1 -> MATLAB Function/1(X)
  MATLAB Function/1(H) -> C/1
  Constant/1 -> MATLAB Function/5(a)
  u/1 -> Demux/1
  Demux/1 -> MATLAB Function/2(x_ac)
  Demux/3 -> MATLAB Function/4(psi_ac)
  Demux/2 -> MATLAB Function/3(y_ac)
  Constant1/1 -> MATLAB Function/6(delta_h)

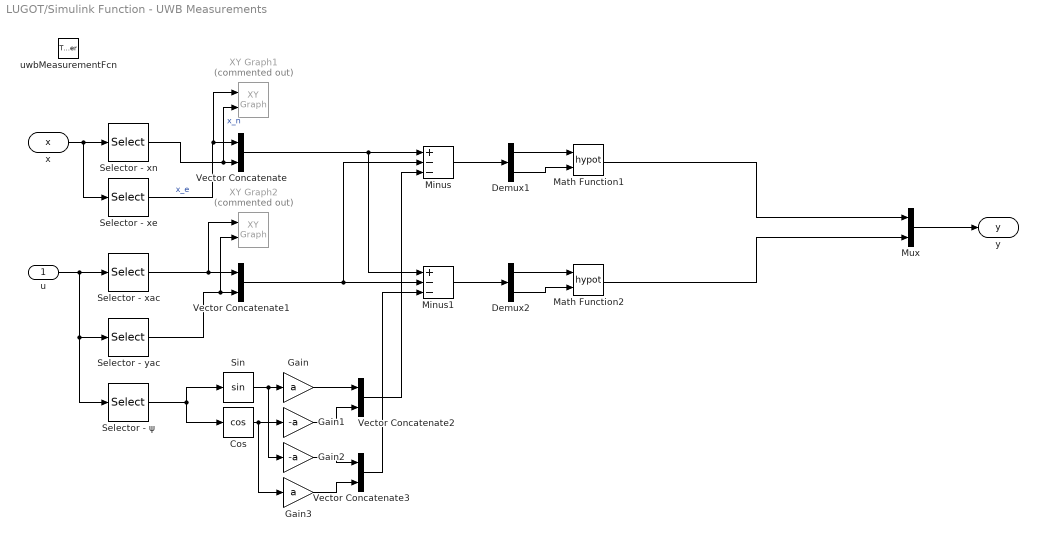
== system LUGOT/Simulink Function - UWB Measurements ==
  u : Inport
  uwbMeasurementFcn : TriggerPort  TriggerType=function-call  IsSimulinkFunction=on  FunctionName=uwbMeasurementFcn  VariantControl=Variant
  Cos : Trigonometry  Operator=cos
  Demux1 : Demux  Outputs=2
  Demux2 : Demux  Outputs=2
  Gain : Gain  Gain=a
  Gain1 : Gain  Gain=-a
  Gain2 : Gain  Gain=-a
  Gain3 : Gain  Gain=a
  Math Function1 : Math  Operator=hypot  SignedPower=on  SaturateOnIntegerOverflow=on
  Math Function2 : Math  Operator=hypot  SignedPower=on  SaturateOnIntegerOverflow=on
  Minus : Sum  Inputs=+--
  Minus1 : Sum  Inputs=+--
  Mux : Mux  Inputs=2
  Selector - xac : Selector  InputPortWidth=3  IndexOptions=Index vector (dialog)  Indices=1  OutputSizes=1
  Selector - xe : Selector  InputPortWidth=4  IndexOptions=Index vector (dialog)  Indices=1  OutputSizes=1
  Selector - xn : Selector  InputPortWidth=4  IndexOptions=Index vector (dialog)  Indices=2  OutputSizes=1
  Selector - yac : Selector  InputPortWidth=3  IndexOptions=Index vector (dialog)  Indices=2  OutputSizes=1
  Selector - ψ : Selector  InputPortWidth=3  IndexOptions=Index vector (dialog)  Indices=3  OutputSizes=1
  Sin : Trigonometry
  Vector Concatenate{,1..3} (4 alike) : Concatenate
  XY Graph1 : simulink/Sinks/XY Graph  Commented=on  xmin=0  xmax=220  ymin=-17  ymax=34  st=-1
  XY Graph2 : simulink/Sinks/XY Graph  Commented=on  xmin=0  xmax=220  ymin=-17  ymax=34  st=-1
  x : ArgIn  DisableCoverage=on  PortDimensions=4  ArgumentName=x
  y : ArgOut  DisableCoverage=on  PortDimensions=2  ArgumentName=y
  wires:
  Math Function2/1 -> Mux/2
  Math Function1/1 -> Mux/1
  Selector - xe/1 -> XY Graph1/1, Vector Concatenate/1  "x_e"
  Selector - xn/1 -> XY Graph1/2, Vector Concatenate/2  "x_n"
  x/1 -> Selector - xn/1, Selector - xe/1
  u/1 -> Selector - ψ/1, Selector - yac/1, Selector - xac/1
  Selector - xac/1 -> XY Graph2/1, Vector Concatenate1/1
  Selector - yac/1 -> XY Graph2/2, Vector Concatenate1/2
  Selector - ψ/1 -> Sin/1, Cos/1
  Gain/1 -> Vector Concatenate2/1
  Gain1/1 -> Vector Concatenate2/2
  Gain3/1 -> Vector Concatenate3/2
  Sin/1 -> Gain2/1, Gain/1
  Cos/1 -> Gain3/1, Gain1/1
  Gain2/1 -> Vector Concatenate3/1
  Vector Concatenate/1 -> Minus1/1, Minus/1
  Vector Concatenate1/1 -> Minus/2, Minus1/2
  Vector Concatenate2/1 -> Minus/3
  Vector Concatenate3/1 -> Minus1/3
  Minus/1 -> Demux1/1
  Demux1/1 -> Math Function1/1
  Demux1/2 -> Math Function1/2
  Demux2/2 -> Math Function2/2
  Demux2/1 -> Math Function2/1
  Minus1/1 -> Demux2/1
  Mux/1 -> y/1

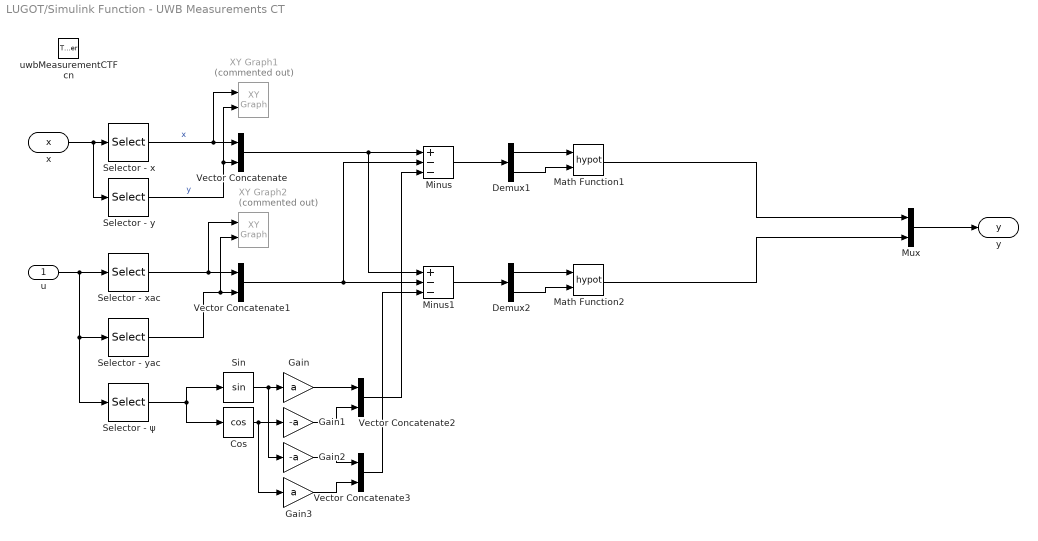
== system LUGOT/Simulink Function - UWB Measurements CT ==
  u : Inport
  uwbMeasurementCTFcn : TriggerPort  TriggerType=function-call  IsSimulinkFunction=on  FunctionName=uwbMeasurementCTFcn  VariantControl=Variant
  Cos : Trigonometry  Operator=cos
  Demux1 : Demux  Outputs=2
  Demux2 : Demux  Outputs=2
  Gain : Gain  Gain=a
  Gain1 : Gain  Gain=-a
  Gain2 : Gain  Gain=-a
  Gain3 : Gain  Gain=a
  Math Function1 : Math  Operator=hypot  SignedPower=on  SaturateOnIntegerOverflow=on
  Math Function2 : Math  Operator=hypot  SignedPower=on  SaturateOnIntegerOverflow=on
  Minus : Sum  Inputs=+--
  Minus1 : Sum  Inputs=+--
  Mux : Mux  Inputs=2
  Selector - x : Selector  InputPortWidth=5  IndexOptions=Index vector (dialog)  Indices=1  OutputSizes=1
  Selector - xac : Selector  InputPortWidth=3  IndexOptions=Index vector (dialog)  Indices=1  OutputSizes=1
  Selector - y : Selector  InputPortWidth=5  IndexOptions=Index vector (dialog)  Indices=3  OutputSizes=1
  Selector - yac : Selector  InputPortWidth=3  IndexOptions=Index vector (dialog)  Indices=2  OutputSizes=1
  Selector - ψ : Selector  InputPortWidth=3  IndexOptions=Index vector (dialog)  Indices=3  OutputSizes=1
  Sin : Trigonometry
  Vector Concatenate{,1..3} (4 alike) : Concatenate
  XY Graph1 : simulink/Sinks/XY Graph  Commented=on  xmin=0  xmax=220  ymin=-17  ymax=34  st=-1
  XY Graph2 : simulink/Sinks/XY Graph  Commented=on  xmin=0  xmax=220  ymin=-17  ymax=34  st=-1
  x : ArgIn  DisableCoverage=on  PortDimensions=5  ArgumentName=x
  y : ArgOut  DisableCoverage=on  PortDimensions=2  ArgumentName=y
  wires:
  Mux/1 -> y/1
  Minus1/1 -> Demux2/1
  Demux2/1 -> Math Function2/1
  Demux2/2 -> Math Function2/2
  Demux1/2 -> Math Function1/2
  Demux1/1 -> Math Function1/1
  Minus/1 -> Demux1/1
  Vector Concatenate3/1 -> Minus1/3
  Vector Concatenate2/1 -> Minus/3
  Vector Concatenate1/1 -> Minus1/2, Minus/2
  Vector Concatenate/1 -> Minus/1, Minus1/1
  Gain2/1 -> Vector Concatenate3/1
  Cos/1 -> Gain1/1, Gain3/1
  Sin/1 -> Gain/1, Gain2/1
  Gain3/1 -> Vector Concatenate3/2
  Gain1/1 -> Vector Concatenate2/2
  Gain/1 -> Vector Concatenate2/1
  Selector - ψ/1 -> Cos/1, Sin/1
  Selector - yac/1 -> Vector Concatenate1/2, XY Graph2/2
  Selector - xac/1 -> Vector Concatenate1/1, XY Graph2/1
  u/1 -> Selector - xac/1, Selector - yac/1, Selector - ψ/1
  x/1 -> Selector - x/1, Selector - y/1
  Selector - y/1 -> Vector Concatenate/2, XY Graph1/2  "y"
  Selector - x/1 -> Vector Concatenate/1, XY Graph1/1  "x"
  Math Function1/1 -> Mux/1
  Math Function2/1 -> Mux/2
